simulink model "BE_Trotinette"  (R2020a)
settings: Solver=VariableStepAuto  StartTime=0.0  StopTime=0.01  RelTol=1e-3
libraries: cstblocks x3
settings Model: Creator=menendez  LastModifiedBy=menendez

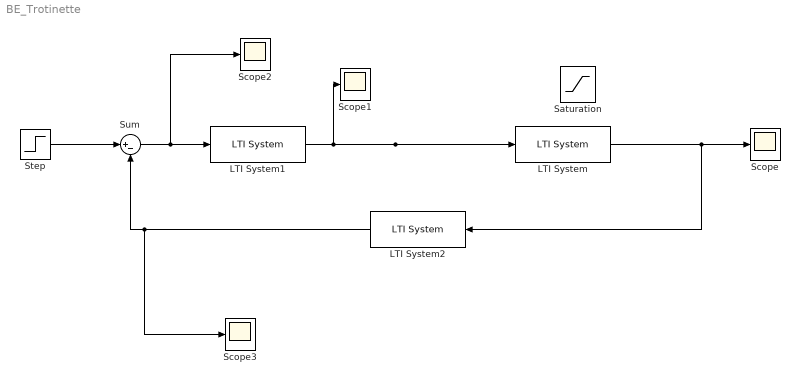
== system BE_Trotinette ==
  LTI System : cstblocks/LTI System  sys=G  IC=[]
  LTI System1 : cstblocks/LTI System  sys=C  IC=[]
  LTI System2 : cstblocks/LTI System  sys=F  IC=[]
  Saturation : Saturate  UpperLimit=0.21
  Scope{,1..3} (4 alike) : Scope
  Step : Step  Time=0  After=0.5  SampleTime=0
  Sum : Sum  Inputs=|+-
  wires:
  Sum/1 -> Scope2/1, LTI System1/1
  Step/1 -> Sum/1
  LTI System2/1 -> Scope3/1, Sum/2
  LTI System/1 -> Scope/1, LTI System2/1
  LTI System1/1 -> LTI System/1, Scope1/1
